simulink model "move_index_test"  (R2020b)
settings: Solver=FixedStepDiscrete  StartTime=0.0  StopTime=10.0  FixedStep=0.1  RelTol=1e-3
values from neighbouring files (symbols this model uses):
  kRollOverAdjustment = int16(-1)    [move_index_params.m]
undefined symbols (not defined in the file or in its folder): kContainerLength, kFirstContainerIndex, kLastContainerIndex
libraries: simulink x1
settings Model: Creator=rsub  LastModifiedBy=rsub

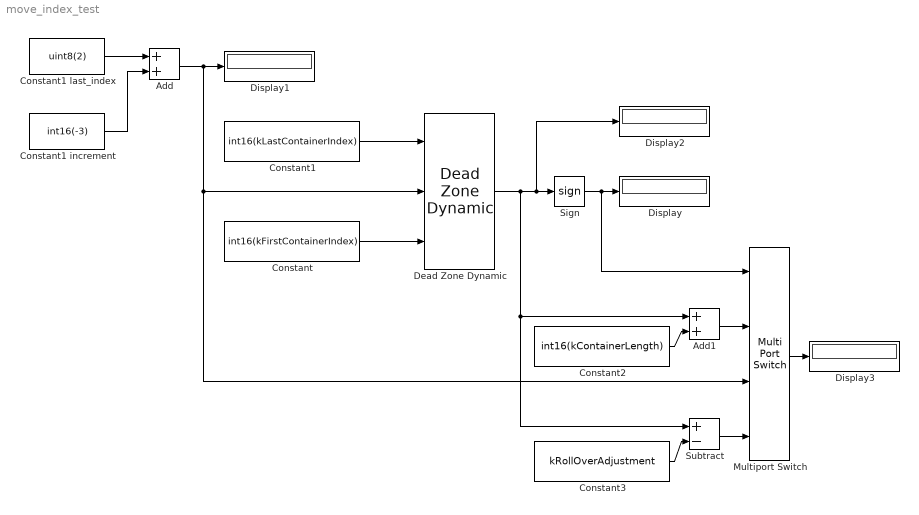
== system move_index_test ==
  Add : Sum  OutDataTypeStr=int16
  Add1 : Sum
  Constant : Constant  Value=int16(kFirstContainerIndex)
  Constant1 : Constant  Value=int16(kLastContainerIndex)
  Constant1 increment : Constant  Value=int16(-3)
  Constant1 last_index : Constant  Value=uint8(2)
  Constant2 : Constant  Value=int16(kContainerLength)
  Constant3 : Constant  Value=kRollOverAdjustment
  Dead Zone Dynamic : simulink/Discontinuities/Dead Zone Dynamic
      settings: SourceProductBaseCode=SL
  Display{,1..3} (4 alike) : Display
  Multiport Switch : MultiPortSwitch  DataPortOrder=Specify indices  DataPortIndices={-1,0,1}
  Sign : Signum
  Subtract : Sum  Inputs=+-
  wires:
  Constant1 last_index/1 -> Add/1
  Constant1 increment/1 -> Add/2
  Add/1 -> Multiport Switch/3, Dead Zone Dynamic/2, Display1/1
  Constant/1 -> Dead Zone Dynamic/3
  Constant1/1 -> Dead Zone Dynamic/1
  Dead Zone Dynamic/1 -> Subtract/1, Add1/1, Display2/1, Sign/1
  Sign/1 -> Multiport Switch/1, Display/1
  Add1/1 -> Multiport Switch/2
  Constant2/1 -> Add1/2
  Multiport Switch/1 -> Display3/1
  Subtract/1 -> Multiport Switch/4
  Constant3/1 -> Subtract/2
